simulink model "Ejer3P2"  (R2024b)
settings: Solver=VariableStepAuto  StartTime=0.0  StopTime=10.0  RelTol=1e-3
settings Model: Creator=lopez  LastModifiedBy=lopez

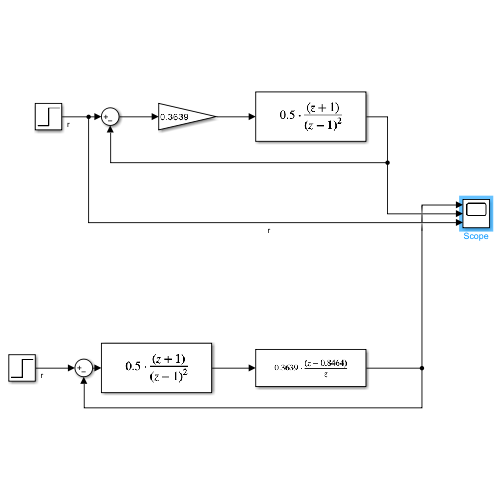
[thumbnail: Simulink's stored preview of the top-level diagram]
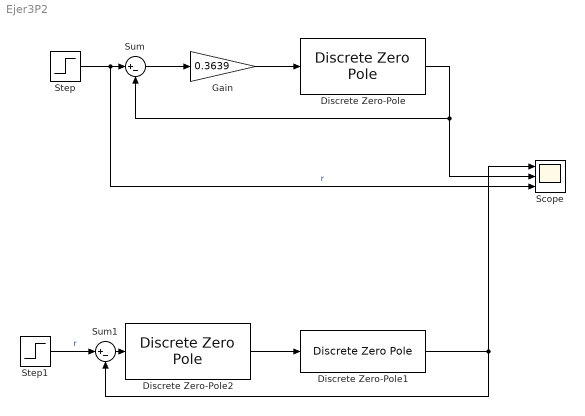
== system Ejer3P2 ==
  Discrete Zero-Pole : DiscreteZeroPole  Zeros=[-1]  Poles=[1 1]  Gain=0.5  SampleTime=0.1
  Discrete Zero-Pole1 : DiscreteZeroPole  Zeros=[0.8464]  Poles=[0]  Gain=0.3639  SampleTime=-1
  Discrete Zero-Pole2 : DiscreteZeroPole  Zeros=[-1]  Poles=[1 1]  Gain=0.5  SampleTime=0.1
  Gain : Gain  Gain=0.3639
  Scope : Scope  NumInputPorts=3
  Step : Step  Time=0  SampleTime=0
  Step1 : Step  Time=0  SampleTime=0
  Sum : Sum  Inputs=|+-
  Sum1 : Sum  Inputs=|+-
  wires:
  Step/1 -> Scope/3, Sum/1  "r"
  Step1/1 -> Sum1/1  "r"
  Discrete Zero-Pole1/1 -> Sum1/2, Scope/1
  Sum1/1 -> Discrete Zero-Pole2/1
  Discrete Zero-Pole2/1 -> Discrete Zero-Pole1/1
  Sum/1 -> Gain/1
  Discrete Zero-Pole/1 -> Scope/2, Sum/2
  Gain/1 -> Discrete Zero-Pole/1
